simulink model "IOControls"  (R2019b)
settings: configuration reference "ConfigSet_IOControls_Reference" (kept outside this file)
model workspace (MAT data in the model file):
  SampleTime = 0.05
libraries: IOStateMachinesLib x274, SignalGeneratorsLib x1, simulink x1
(part 1 of 10)
settings Model: Creator=lonkaran  LastModifiedBy=bnadpurohit
settings ConfigSetRef: SourceName=ConfigSet_IOControls_Reference  SourceLocation=Base Workspace

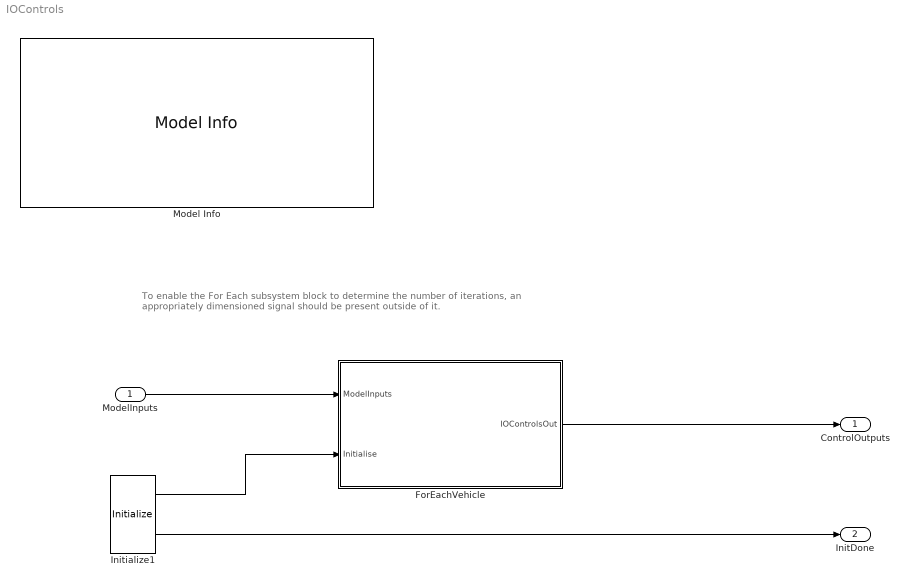
== system IOControls ==
  note: To enable the For Each subsystem block to determine the number of iterations,
      | an appropriately dimensioned signal should be present outside of it.
  ModelInputs : Inport  OutDataTypeStr=Bus: BD_IOControls_In_Vehicle  PortDimensions=MaxVehicles  BusOutputAsStruct=on
  ForEachVehicle : Subsystem  TreatAsAtomicUnit=on
  Initialize1 : SignalGeneratorsLib/Initialize  InitTime=2  SampleTime=0.1
      settings: SourceProductName=Signal Generators
  Model Info : simulink/Model-Wide Utilities/Model Info  Frame=on  DisplayStringWithTags=Model Info\nTemplate Name: IOControlsTemplate\nTemplate Model version number: 1.61\nLast modification date: Thu Jan 23 11:29:17 2020\nModel description:\n\nThis model was created on : %<LastModificationDate> \n automatically by the create_io_controls script using the data available from \nBEML_EMU Model IO.csv  HorizontalTextAlignment=Left  LeftAlignmentValue=0.02
  ControlOutputs : Outport  OutDataTypeStr=Bus: BD_IOControls_Out_Vehicle  VectorParamsAs1DForOutWhenUnconnected=off  BusOutputAsStruct=on
  InitDone : Outport  Port=2  VectorParamsAs1DForOutWhenUnconnected=off
  wires:
  ForEachVehicle/1(IOControlsOut) -> ControlOutputs/1
  ModelInputs/1 -> ForEachVehicle/1(ModelInputs)
  Initialize1/1 -> ForEachVehicle/2(Initialise)
  Initialize1/2 -> InitDone/1

== system IOControls/ForEachVehicle ==
  note: Process inputs from each panel
  ModelInputs : Inport  Partition=on  PartitionDimension=1  PartitionWidth=1  PartitionOffset=0
  Initialise : Inport  Port=2
  For Each : ForEach  DisableCoverage=on
  IOControls : Subsystem
  OutputMapper : Subsystem
  IOControlsOut : Outport  ConcatenationDimension=1  VectorParamsAs1DForOutWhenUnconnected=off
  wires:
  OutputMapper/1(IOControlsOut) -> IOControlsOut/1
  IOControls/1(TierControlsInputs) -> OutputMapper/1(TierControlsInputs)
  ModelInputs/1 -> IOControls/1(ModelInputs)
  Initialise/1 -> IOControls/2(Initialise)
  IOControls/2(TierControlsMCBTrip) -> OutputMapper/2(TierControlsMCBTrip)

== system IOControls/ForEachVehicle/IOControls ==
  ModelInputs : Inport
  Initialise : Inport  Port=2
  BC_Inputs : BusCreator  Inputs=2
  BC_MCBTrip : BusCreator  Inputs=2
  CabControl : Subsystem
  Non-CabControl : Subsystem
  TierControlsInputs : Outport  VectorParamsAs1DForOutWhenUnconnected=off
  TierControlsMCBTrip : Outport  Port=2  VectorParamsAs1DForOutWhenUnconnected=off
  wires:
  BC_Inputs/1 -> TierControlsInputs/1
  BC_MCBTrip/1 -> TierControlsMCBTrip/1
  ModelInputs/1 -> CabControl/1(ModelInputs), Non-CabControl/1(ModelInputs)
  Initialise/1 -> CabControl/2(Initialise), Non-CabControl/2(Initialise)
  CabControl/1(TierControlsInputs) -> BC_Inputs/1
  CabControl/2(TierControlsMCBTrip) -> BC_MCBTrip/1
  Non-CabControl/1(TierControlsInputs) -> BC_Inputs/2
  Non-CabControl/2(TierControlsMCBTrip) -> BC_MCBTrip/2

== system IOControls/ForEachVehicle/OutputMapper ==
  TierControlsInputs : Inport
  TierControlsMCBTrip : Inport  Port=2
  BC_IOControlsOut : BusCreator  Inputs=3  OutDataTypeStr=Bus: BD_IOControls_Out_Vehicle  NonVirtualBus=on
  BS_Inputs : BusSelector  OutputSignals=CabControl.DriverDesk.OperatingPanel1.EmergencyBrakePB,CabControl.DriverDesk.OperatingPanel1.HornPB,CabControl.DriverDesk.OperatingPanel1.CabConsoleLightPB,CabControl.DriverDesk.OperatingPanel1.DoorProvenLoopCutoutPB,CabControl.DriverDesk.OperatingPanel1.LeftDoorClosePBOperatingPanel1,CabControl.DriverDesk.OperatingPanel1.RightDoorClosePBOperatingPanel1,CabControl.DriverDesk.OperatingPanel1.LeftDoorOpenPBOperatingPanel1,CabControl.DriverDesk.OperatingPanel1.RightDoorOpenPBOperatingPanel1,CabControl.DriverDesk.OperatingPanel1.CabMainLightPB,CabControl.DriverDesk.OperatingPanel1.ParkingBrakeOnSwitch,CabControl.DriverDesk.OperatingPanel1.ParkingBrakeOffSwitch,CabControl.DriverDesk.OperatingPanel1.DoorCloseAnnouncementPB,CabControl.DriverDesk.OperatingPanel3.ROSPB,CabControl.DriverDesk.OperatingPanel3.UTOPB,CabControl.DriverDesk.OperatingPanel3.ATOStartPB,CabControl.DriverDesk.OperatingPanel3.EmergencyBrakeResetPB,CabControl.DriverDesk.MasterController.ControlKey,CabControl.DriverDesk.MasterController.ModeSelector,CabControl.DriverDesk.MasterController.MasterControllerHandle,CabControl.DriverDesk.MasterController.DeadmanSafetyDevice,CabControl.DriverDeskLeft.OperatingPanel2.CallOnLightPB,CabControl.DriverDeskLeft.OperatingPanel2.VCBOpenPB,CabControl.DriverDeskLeft.OperatingPanel2.WiperSelectionSwitch,CabControl.DriverDeskLeft.OperatingPanel2.WiperPump,CabControl.DriverDeskLeft.OperatingPanel2.LIMPHomePB,CabControl.DriverDeskLeft.OperatingPanel2.PowerOffPB,CabControl.DriverDeskLeft.OperatingPanel2.PantoDownPB,CabControl.DriverDeskLeft.OperatingPanel2.VCBClosePB,CabControl.DriverDeskLeft.OperatingPanel2.LeftDoorOpenPBOperatingPanel2,CabControl.DriverDeskLeft.OperatingPanel2.LeftDoorOpenPB1OperatingPanel2,CabControl.DriverDeskLeft.OperatingPanel2.LeftDoorClosePBOperatingPanel2,CabControl.DriverDeskLeft.OperatingPanel2.PantoUpPB,CabControl.DriverDeskLeft.OperatingPanel2.SafetyCutoutSS,CabControl.DriverDeskLeft.OperatingPanel2.BrakeLoopCutoutSS,CabControl.DriverDeskLeft.OperatingPanel2.PantoSelector,CabControl.DriverDeskLeft.OperatingPanel2.DeadmanBypassSwitch,CabControl.DriverDeskLeft.OperatingPanel2.HeadLightSwitch,CabControl.DriverDeskRight.OperatingPanel5.UncouplePB,CabControl.DriverDeskRight.OperatingPanel5.FlasherLightPB,CabControl.DriverDeskRight.OperatingPanel5.FloodLightPB,CabControl.DriverDeskRight.OperatingPanel5.BatteryResetPB,CabControl.DriverDeskRight.OperatingPanel5.RightDoorOpenPBOperatingPanel5,CabControl.DriverDeskRight.OperatingPanel5.RightDoorOpenPB1OperatingPanel5,CabControl.DriverDeskRight.OperatingPanel5.RightDoorClosePBOperatingPanel5,CabControl.DriverDeskRight.OperatingPanel5.DoorProvenLoopOutputSwitch,CabControl.DriverDeskRight.OperatingPanel5.LampTestPB,CabControl.DriverDeskRight.OperatingPanel5.WFLTestPB,CabControl.DriverDeskRight.OperatingPanel5.WiperControlSwitch,CabControl.DriverDeskRight.OperatingPanel5.EmergencyStopPB,CabControl.DriverDeskRight.OperatingPanel5.HoldDoorCloseBypassSS,CabControl.DriverDeskRight.OperatingPanel5.CabBoosterFanSS,CabControl.DriverDeskRight.OperatingPanel5.EmergencyBrakePBBypassSS,CabControl.DriversSideCovingPanel.CabEEDLeft,CabControl.Non-driversSideCovingPanel.CabEEDRight,CabControl.EmergencyDoor.SafetyCover,CabControl.EmergencyDoor.DummyCover,CabControl.EmergencyDoor.RampCoverLockingLever,CabControl.EmergencyDoor.RampCover,CabControl.EmergencyDoor.RampHandle,CabControl.EmergencyDoor.RampEndSupport,CabControl.EmergencyDoor.RampMiddleSupport,CabControl.EmergencyDoor.WinderHandlesAccessCover,CabControl.EmergencyDoor.LargeHandle,CabControl.EmergencyDoor.RampWinder,CabControl.EmergencyDoor.SmallHandle,CabControl.EmergencyDoor.EmergencyDoorGasSpring,CabControl.EmergencyDoor.DoorWinder,Non-CabControl.CircuitBreakersofEDB.EBLR2CB,Non-CabControl.CircuitBreakersofEDB.EBMVCB,Non-CabControl.CircuitBreakersofEDB.EDCB,Non-CabControl.CircuitBreakersofEDB.ELCB1,Non-CabControl.CircuitBreakersofEDB.ELCB2,Non-CabControl.CircuitBreakersofEDB.ERCB,Non-CabControl.CircuitBreakersofEDB.HCB,Non-CabControl.CircuitBreakersofEDB.HLLCB,Non-CabControl.CircuitBreakersofEDB.HLRCB,Non-CabControl.CircuitBreakersofEDB.ILCB1,Non-CabControl.CircuitBreakersofEDB.ILCB2,Non-CabControl.CircuitBreakersofEDB.LDICB,Non-CabControl.CircuitBreakersofEDB.LDLCB,Non-CabControl.CircuitBreakersofEDB.LDRCB,Non-CabControl.CircuitBreakersofEDB.MLCB,Non-CabControl.CircuitBreakersofEDB.MMCB,Non-CabControl.CircuitBreakersofEDB.NBCB,Non-CabControl.CircuitBreakersofEDB.NVICB,Non-CabControl.CircuitBreakersofEDB.OCCB1,Non-CabControl.CircuitBreakersofEDB.OCCB2,Non-CabControl.CircuitBreakersofEDB.ODDCB,Non-CabControl.CircuitBreakersofEDB.PBCB,Non-CabControl.CircuitBreakersofEDB.PISCB1,Non-CabControl.CircuitBreakersofEDB.PISCB2,Non-CabControl.CircuitBreakersofEDB.POCB,Non-CabControl.CircuitBreakersofEDB.PPU1CB,Non-CabControl.CircuitBreakersofEDB.PPU2CB,Non-CabControl.CircuitBreakersofEDB.PPU3CB,Non-CabControl.CircuitBreakersofEDB.RIO1CB,Non-CabControl.CircuitBreakersofEDB.RIO2CB,Non-CabControl.CircuitBreakersofEDB.SIOCB1,Non-CabControl.CircuitBreakersofEDB.SIOCB2,Non-CabControl.CircuitBreakersofEDB.SSICB,Non-CabControl.CircuitBreakersofEDB.TBCCB1,Non-CabControl.CircuitBreakersofEDB.TBCCB2,Non-CabControl.CircuitBreakersofEDB.TBNCB,Non-CabControl.CircuitBreakersofEDB.TDICB,Non-CabControl.CircuitBreakersofEDB.TLLCB,Non-CabControl.CircuitBreakersofEDB.TLRCB,Non-CabControl.CircuitBreakersofEDB.TRIVCB,Non-CabControl.CircuitBreakersofEDB.TVDUCB,Non-CabControl.CircuitBreakersofEDB.TWVCB,Non-CabControl.CircuitBreakersofEDB.VCCBOrUCCB,Non-CabControl.CircuitBreakersofEDB.VCBCCB,Non-CabControl.CircuitBreakersofEDB.VIO1CB,Non-CabControl.CircuitBreakersofEDB.VIO2CB,Non-CabControl.CircuitBreakersofEDB.WFLCB,Non-CabControl.CircuitBreakersofEDB.WIFICB,Non-CabControl.CircuitBreakersofEDB.WWCB,Non-CabControl.CircuitBreakersofEDB.BECUCB1,Non-CabControl.CircuitBreakersofEDB.BECUCB2,Non-CabControl.CircuitBreakersofEDB.BECUCB3,Non-CabControl.CircuitBreakersofEDB.RSACB,Non-CabControl.CircuitBreakersofEDB.CMCCB,Non-CabControl.CircuitBreakersofEDB.CILCB,Non-CabControl.CircuitBreakersofEDB.CICB,Non-CabControl.CircuitBreakersofEDB.CELCB,Non-CabControl.CircuitBreakersofEDB.CECB,Non-CabControl.CircuitBreakersofEDB.CDUCB,Non-CabControl.CircuitBreakersofEDB.CCNVIO1CB,Non-CabControl.CircuitBreakersofEDB.CBTCCB1,Non-CabControl.CircuitBreakersofEDB.CBFCCB,Non-CabControl.CircuitBreakersofEDB.CBFCB,Non-CabControl.CircuitBreakersofEDB.C1CB,Non-CabControl.CircuitBreakersofEDB.BLCB,Non-CabControl.CircuitBreakersofEDB.ZVBACB,Non-CabControl.CircuitBreakersofEDB.EBLR1CB,Non-CabControl.CircuitBreakersofEDB.DRCB,Non-CabControl.CircuitBreakersofEDB.DPLCB,Non-CabControl.CircuitBreakersofEDB.DMICB,Non-CabControl.CircuitBreakersofEDB.DLCB,Non-CabControl.CircuitBreakersofEDB.DIOCB2,Non-CabControl.CircuitBreakersofEDB.DIOCB1,Non-CabControl.CircuitBreakersofEDB.CSCCB,Non-CabControl.CircuitBreakersofEDB.CSBCB,Non-CabControl.CircuitBreakersofEDB.CSACB,Non-CabControl.CircuitBreakersofEDB.CRSBCB,Non-CabControl.CircuitBreakersofEDB.SOCB2,Non-CabControl.CircuitBreakersofEDB.SOCB1,Non-CabControl.CircuitBreakersofEDB.MSOCB5,Non-CabControl.CircuitBreakersofEDB.MSOCB4,Non-CabControl.CircuitBreakersofEDB.MSOCB3,Non-CabControl.CircuitBreakersofEDB.MSOCB2,Non-CabControl.CircuitBreakersofEDB.MSOCB1,Non-CabControl.CircuitBreakersofEDB.HVAC1,Non-CabControl.CircuitBreakersofEDB.SAC2CCB,Non-CabControl.CircuitBreakersofEDB.HVAC2,Non-CabControl.CircuitBreakersofEDB.SAC1CCB,Non-CabControl.CircuitBreakersofEDB.CMCB,Non-CabControl.CircuitBreakersofEDB.AC2CB,Non-CabControl.CircuitBreakersofEDB.AC1CB,Non-CabControl.CircuitBreakersofEDB.FDSCB,Non-CabControl.CircuitBreakersofEDB.BCBCB,Non-CabControl.CircuitBreakersofEDB.ERVRCB1,Non-CabControl.CircuitBreakersofEDB.ERVRCB2,Non-CabControl.CircuitBreakersofEDB.ESKCB,Non-CabControl.CircuitBreakersofEDB.HMCB,Non-CabControl.CircuitBreakersofEDB.SP1CB,Non-CabControl.CircuitBreakersofEDB.SP2CB,Non-CabControl.CircuitBreakersofEDB.SP3CB,Non-CabControl.CircuitBreakersofEDB.SP4CB,Non-CabControl.CircuitBreakersofEDB.SP5CB,Non-CabControl.CircuitBreakersofEDB.SPCB6,Non-CabControl.CircuitBreakersofEDB.SPCB7,Non-CabControl.CircuitBreakersofEDB.SPCB8,Non-CabControl.CircuitBreakersofEDB.RPTCB,Non-CabControl.CircuitBreakersofEDB.TERCB1,Non-CabControl.CircuitBreakersofEDB.TERCB2,Non-CabControl.CircuitBreakersofEDB.SPSW,Non-CabControl.CircuitBreakersofEDB.SPPB,Non-CabControl.CircuitBreakersofEDB.APSCB,Non-CabControl.CircuitBreakersofEDB.APSICB,Non-CabControl.CircuitBreakersofEDB.BCGCB,Non-CabControl.CircuitBreakersofEDB.DSCB,Non-CabControl.CircuitBreakersofEDB.MTBMCCB,Non-CabControl.CircuitBreakersofEDB.PADCB,Non-CabControl.CircuitBreakersofEDB.PANCB,Non-CabControl.CircuitBreakersofEDB.SSCB,Non-CabControl.CircuitBreakersofEDB.PTCB,Non-CabControl.CircuitBreakersofEDB.VCBCB,Non-CabControl.CircuitBreakersofEDB.SP12CB,Non-CabControl.CircuitBreakersofEDB.MTBM1CB,Non-CabControl.CircuitBreakersofEDB.MTBM2CB,Non-CabControl.CircuitBreakersofEDB.SP11CB,Non-CabControl.CircuitBreakersofEDB.SP6CB,Non-CabControl.CircuitBreakersofEDB.MTOPCB,Non-CabControl.CircuitBreakersofEDB.ORDCOS,Non-CabControl.CircuitBreakersofEDB.ADDCOS,Non-CabControl.InteriorDoorControls.LeftDoor1DCUCB,Non-CabControl.InteriorDoorControls.LeftDoor2DCUCB,Non-CabControl.InteriorDoorControls.LeftDoor3DCUCB,Non-CabControl.InteriorDoorControls.LeftDoor4DCUCB,Non-CabControl.InteriorDoorControls.RightDoor1DCUCB,Non-CabControl.InteriorDoorControls.RightDoor2DCUCB,Non-CabControl.InteriorDoorControls.RightDoor3DCUCB,Non-CabControl.InteriorDoorControls.RightDoor4DCUCB,Non-CabControl.InteriorDoorControls.LeftDoor1Coving,Non-CabControl.InteriorDoorControls.LeftDoor2Coving,Non-CabControl.InteriorDoorControls.LeftDoor3Coving,Non-CabControl.InteriorDoorControls.LeftDoor4Coving,Non-CabControl.InteriorDoorControls.RightDoor1Coving,Non-CabControl.InteriorDoorControls.RightDoor2Coving,Non-CabControl.InteriorDoorControls.RightDoor3Coving,Non-CabControl.InteriorDoorControls.RightDoor4Coving,Non-CabControl.InteriorDoorControls.LeftDoor1EED,Non-CabControl.InteriorDoorControls.LeftDoor2EED,Non-CabControl.InteriorDoorControls.LeftDoor3EED,Non-CabControl.InteriorDoorControls.LeftDoor4EED,Non-CabControl.InteriorDoorControls.RightDoor1EED,Non-CabControl.InteriorDoorControls.RightDoor2EED,Non-CabControl.InteriorDoorControls.RightDoor3EED,Non-CabControl.InteriorDoorControls.RightDoor4EED,Non-CabControl.InteriorDoorControls.LeftDoor1ManualClose,Non-CabControl.InteriorDoorControls.LeftDoor2ManualClose,Non-CabControl.InteriorDoorControls.LeftDoor3ManualClose,Non-CabControl.InteriorDoorControls.LeftDoor4ManualClose,Non-CabControl.InteriorDoorControls.RightDoor1ManualClose,Non-CabControl.InteriorDoorControls.RightDoor2ManualClose,Non-CabControl.InteriorDoorControls.RightDoor3ManualClose,Non-CabControl.InteriorDoorControls.RightDoor4ManualClose,Non-CabControl.InteriorDoorControls.LeftDoor1ManualOpen,Non-CabControl.InteriorDoorControls.LeftDoor2ManualOpen,Non-CabControl.InteriorDoorControls.LeftDoor3ManualOpen,Non-CabControl.InteriorDoorControls.LeftDoor4ManualOpen,Non-CabControl.InteriorDoorControls.RightDoor1ManualOpen,Non-CabControl.InteriorDoorControls.RightDoor2ManualOpen,Non-CabControl.InteriorDoorControls.RightDoor3ManualOpen,Non-CabControl.InteriorDoorControls.RightDoor4ManualOpen,Non-CabControl.InteriorDoorControls.LeftDoor1Lockout,Non-CabControl.InteriorDoorControls.LeftDoor2Lockout,Non-CabControl.InteriorDoorControls.LeftDoor3Lockout,Non-CabControl.InteriorDoorControls.LeftDoor4Lockout,Non-CabControl.InteriorDoorControls.RightDoor1Lockout,Non-CabControl.InteriorDoorControls.RightDoor2Lockout,Non-CabControl.InteriorDoorControls.RightDoor3Lockout,Non-CabControl.InteriorDoorControls.RightDoor4Lockout,Non-CabControl.ExteriorDoorControls.LeftDoorEADCover,Non-CabControl.ExteriorDoorControls.RightDoorEADCover,Non-CabControl.ExteriorDoorControls.LeftDoorEAD,Non-CabControl.ExteriorDoorControls.RightDoorEAD,Non-CabControl.PneumaticControls.ParkBrakeIsolationCockBogie1,Non-CabControl.PneumaticControls.ParkBrakeIsolationCockBogie2,Non-CabControl.PneumaticControls.MRIsolationCock,Non-CabControl.PneumaticControls.UncouplingCock,Non-CabControl.PneumaticControls.Horn1IsolationCock,Non-CabControl.PneumaticControls.Horn2IsolationCock,Non-CabControl.PneumaticControls.MREPIsolationCockEnd1,Non-CabControl.PneumaticControls.BIC1Inside,Non-CabControl.PneumaticControls.BIC1Outside,Non-CabControl.PneumaticControls.BIC2Inside,Non-CabControl.PneumaticControls.BIC2Outside,Non-CabControl.PneumaticControls.MREPIsolationCockEnd2,Non-CabControl.PneumaticControls.EPIC,Non-CabControl.PneumaticControls.ASCOEnd1,Non-CabControl.PneumaticControls.ASCOEnd2,Non-CabControl.PneumaticControls.ASIsolationCock,Non-CabControl.PneumaticControls.SR,Non-CabControl.PneumaticControls.ParkingBrakeManualReleaseBogie1Handle1,Non-CabControl.PneumaticControls.ParkingBrakeManualReleaseBogie1Handle2,Non-CabControl.PneumaticControls.ParkingBrakeManualReleaseBogie2Handle1,Non-CabControl.PneumaticControls.ParkingBrakeManualReleaseBogie2Handle2,Non-CabControl.PassengerEmergencyControlUnit.PECUPushButton,Non-CabControl.PassengerEmergencyControlUnit.Microphone,Non-CabControl.PassengerEmergencyControlUnit.DriversBackDoor,Non-CabControl.EDBPanel.PantographIsolationCock,Non-CabControl.EDBPanel.VCBIsolationCock,Non-CabControl.EDBPanel.ORDPlunger  OutputAsBus=on
  BS_MCBTrip : BusSelector  OutputSignals=Non-CabControl.CircuitBreakersofEDB.EBLR2CB,Non-CabControl.CircuitBreakersofEDB.EBMVCB,Non-CabControl.CircuitBreakersofEDB.EDCB,Non-CabControl.CircuitBreakersofEDB.ELCB1,Non-CabControl.CircuitBreakersofEDB.ELCB2,Non-CabControl.CircuitBreakersofEDB.ERCB,Non-CabControl.CircuitBreakersofEDB.HCB,Non-CabControl.CircuitBreakersofEDB.HLLCB,Non-CabControl.CircuitBreakersofEDB.HLRCB,Non-CabControl.CircuitBreakersofEDB.ILCB1,Non-CabControl.CircuitBreakersofEDB.ILCB2,Non-CabControl.CircuitBreakersofEDB.LDICB,Non-CabControl.CircuitBreakersofEDB.LDLCB,Non-CabControl.CircuitBreakersofEDB.LDRCB,Non-CabControl.CircuitBreakersofEDB.MLCB,Non-CabControl.CircuitBreakersofEDB.MMCB,Non-CabControl.CircuitBreakersofEDB.NBCB,Non-CabControl.CircuitBreakersofEDB.NVICB,Non-CabControl.CircuitBreakersofEDB.OCCB1,Non-CabControl.CircuitBreakersofEDB.OCCB2,Non-CabControl.CircuitBreakersofEDB.ODDCB,Non-CabControl.CircuitBreakersofEDB.PBCB,Non-CabControl.CircuitBreakersofEDB.PISCB1,Non-CabControl.CircuitBreakersofEDB.PISCB2,Non-CabControl.CircuitBreakersofEDB.POCB,Non-CabControl.CircuitBreakersofEDB.PPU1CB,Non-CabControl.CircuitBreakersofEDB.PPU2CB,Non-CabControl.CircuitBreakersofEDB.PPU3CB,Non-CabControl.CircuitBreakersofEDB.RIO1CB,Non-CabControl.CircuitBreakersofEDB.RIO2CB,Non-CabControl.CircuitBreakersofEDB.SIOCB1,Non-CabControl.CircuitBreakersofEDB.SIOCB2,Non-CabControl.CircuitBreakersofEDB.SSICB,Non-CabControl.CircuitBreakersofEDB.TBCCB1,Non-CabControl.CircuitBreakersofEDB.TBCCB2,Non-CabControl.CircuitBreakersofEDB.TBNCB,Non-CabControl.CircuitBreakersofEDB.TDICB,Non-CabControl.CircuitBreakersofEDB.TLLCB,Non-CabControl.CircuitBreakersofEDB.TLRCB,Non-CabControl.CircuitBreakersofEDB.TRIVCB,Non-CabControl.CircuitBreakersofEDB.TVDUCB,Non-CabControl.CircuitBreakersofEDB.TWVCB,Non-CabControl.CircuitBreakersofEDB.VCCBOrUCCB,Non-CabControl.CircuitBreakersofEDB.VCBCCB,Non-CabControl.CircuitBreakersofEDB.VIO1CB,Non-CabControl.CircuitBreakersofEDB.VIO2CB,Non-CabControl.CircuitBreakersofEDB.WFLCB,Non-CabControl.CircuitBreakersofEDB.WIFICB,Non-CabControl.CircuitBreakersofEDB.WWCB,Non-CabControl.CircuitBreakersofEDB.BECUCB1,Non-CabControl.CircuitBreakersofEDB.BECUCB2,Non-CabControl.CircuitBreakersofEDB.BECUCB3,Non-CabControl.CircuitBreakersofEDB.RSACB,Non-CabControl.CircuitBreakersofEDB.CMCCB,Non-CabControl.CircuitBreakersofEDB.CILCB,Non-CabControl.CircuitBreakersofEDB.CICB,Non-CabControl.CircuitBreakersofEDB.CELCB,Non-CabControl.CircuitBreakersofEDB.CECB,Non-CabControl.CircuitBreakersofEDB.CDUCB,Non-CabControl.CircuitBreakersofEDB.CCNVIO1CB,Non-CabControl.CircuitBreakersofEDB.CBTCCB1,Non-CabControl.CircuitBreakersofEDB.CBFCCB,Non-CabControl.CircuitBreakersofEDB.CBFCB,Non-CabControl.CircuitBreakersofEDB.C1CB,Non-CabControl.CircuitBreakersofEDB.BLCB,Non-CabControl.CircuitBreakersofEDB.ZVBACB,Non-CabControl.CircuitBreakersofEDB.EBLR1CB,Non-CabControl.CircuitBreakersofEDB.DRCB,Non-CabControl.CircuitBreakersofEDB.DPLCB,Non-CabControl.CircuitBreakersofEDB.DMICB,Non-CabControl.CircuitBreakersofEDB.DLCB,Non-CabControl.CircuitBreakersofEDB.DIOCB2,Non-CabControl.CircuitBreakersofEDB.DIOCB1,Non-CabControl.CircuitBreakersofEDB.CSCCB,Non-CabControl.CircuitBreakersofEDB.CSBCB,Non-CabControl.CircuitBreakersofEDB.CSACB,Non-CabControl.CircuitBreakersofEDB.CRSBCB,Non-CabControl.CircuitBreakersofEDB.SOCB2,Non-CabControl.CircuitBreakersofEDB.SOCB1,Non-CabControl.CircuitBreakersofEDB.MSOCB5,Non-CabControl.CircuitBreakersofEDB.MSOCB4,Non-CabControl.CircuitBreakersofEDB.MSOCB3,Non-CabControl.CircuitBreakersofEDB.MSOCB2,Non-CabControl.CircuitBreakersofEDB.MSOCB1,Non-CabControl.CircuitBreakersofEDB.HVAC1,Non-CabControl.CircuitBreakersofEDB.SAC2CCB,Non-CabControl.CircuitBreakersofEDB.HVAC2,Non-CabControl.CircuitBreakersofEDB.SAC1CCB,Non-CabControl.CircuitBreakersofEDB.CMCB,Non-CabControl.CircuitBreakersofEDB.AC2CB,Non-CabControl.CircuitBreakersofEDB.AC1CB,Non-CabControl.CircuitBreakersofEDB.FDSCB,Non-CabControl.CircuitBreakersofEDB.BCBCB,Non-CabControl.CircuitBreakersofEDB.ERVRCB1,Non-CabControl.CircuitBreakersofEDB.ERVRCB2,Non-CabControl.CircuitBreakersofEDB.ESKCB,Non-CabControl.CircuitBreakersofEDB.HMCB,Non-CabControl.CircuitBreakersofEDB.SP1CB,Non-CabControl.CircuitBreakersofEDB.SP2CB,Non-CabControl.CircuitBreakersofEDB.SP3CB,Non-CabControl.CircuitBreakersofEDB.SP4CB,Non-CabControl.CircuitBreakersofEDB.SP5CB,Non-CabControl.CircuitBreakersofEDB.SPCB6,Non-CabControl.CircuitBreakersofEDB.SPCB7,Non-CabControl.CircuitBreakersofEDB.SPCB8,Non-CabControl.CircuitBreakersofEDB.RPTCB,Non-CabControl.CircuitBreakersofEDB.TERCB1,Non-CabControl.CircuitBreakersofEDB.TERCB2,Non-CabControl.CircuitBreakersofEDB.APSCB,Non-CabControl.CircuitBreakersofEDB.APSICB,Non-CabControl.CircuitBreakersofEDB.BCGCB,Non-CabControl.CircuitBreakersofEDB.DSCB,Non-CabControl.CircuitBreakersofEDB.MTBMCCB,Non-CabControl.CircuitBreakersofEDB.PADCB,Non-CabControl.CircuitBreakersofEDB.PANCB,Non-CabControl.CircuitBreakersofEDB.SSCB,Non-CabControl.CircuitBreakersofEDB.PTCB,Non-CabControl.CircuitBreakersofEDB.VCBCB,Non-CabControl.CircuitBreakersofEDB.SP12CB,Non-CabControl.CircuitBreakersofEDB.MTBM1CB,Non-CabControl.CircuitBreakersofEDB.MTBM2CB,Non-CabControl.CircuitBreakersofEDB.SP11CB,Non-CabControl.CircuitBreakersofEDB.SP6CB,Non-CabControl.CircuitBreakersofEDB.MTOPCB,Non-CabControl.InteriorDoorControls.LeftDoor1DCUCB,Non-CabControl.InteriorDoorControls.LeftDoor2DCUCB,Non-CabControl.InteriorDoorControls.LeftDoor3DCUCB,Non-CabControl.InteriorDoorControls.LeftDoor4DCUCB,Non-CabControl.InteriorDoorControls.RightDoor1DCUCB,Non-CabControl.InteriorDoorControls.RightDoor2DCUCB,Non-CabControl.InteriorDoorControls.RightDoor3DCUCB,Non-CabControl.InteriorDoorControls.RightDoor4DCUCB  OutputAsBus=on
  OutputStates : Constant  Value=0  OutDataTypeStr=Bus: BD_IOControls_Out_Vehicle_OutputStates
  IOControlsOut : Outport  VectorParamsAs1DForOutWhenUnconnected=off
  wires:
  BC_IOControlsOut/1 -> IOControlsOut/1  "IOControls"
  OutputStates/1 -> BC_IOControlsOut/3  "OutputStates"
  TierControlsInputs/1 -> BS_Inputs/1
  BS_Inputs/1 -> BC_IOControlsOut/1  "InputStates"
  TierControlsMCBTrip/1 -> BS_MCBTrip/1
  BS_MCBTrip/1 -> BC_IOControlsOut/2  "MCBTripStates"

== system IOControls/ForEachVehicle/IOControls/CabControl ==
  ModelInputs : Inport
  Initialise : Inport  Port=2
  BC_Inputs : BusCreator  Inputs=6
  BC_MCBTrip : BusCreator  Inputs=6
  DriverDesk : Subsystem
  DriverDeskLeft : Subsystem
  DriverDeskRight : Subsystem
  DriversSideCovingPanel : Subsystem
  EmergencyDoor : Subsystem
  Non-driversSideCovingPanel : Subsystem
  TierControlsInputs : Outport  VectorParamsAs1DForOutWhenUnconnected=off
  TierControlsMCBTrip : Outport  Port=2  VectorParamsAs1DForOutWhenUnconnected=off
  wires:
  BC_MCBTrip/1 -> TierControlsMCBTrip/1  "CabControl"
  BC_Inputs/1 -> TierControlsInputs/1  "CabControl"
  ModelInputs/1 -> DriverDesk/1(ModelInputs), DriverDeskLeft/1(ModelInputs), DriverDeskRight/1(ModelInputs), DriversSideCovingPanel/1(ModelInputs), Non-driversSideCovingPanel/1(ModelInputs), EmergencyDoor/1(ModelInputs)
  Initialise/1 -> DriverDesk/2(Initialise), DriverDeskLeft/2(Initialise), DriverDeskRight/2(Initialise), DriversSideCovingPanel/2(Initialise), Non-driversSideCovingPanel/2(Initialise), EmergencyDoor/2(Initialise)
  DriverDesk/1(TierControlsInputs) -> BC_Inputs/1
  DriverDesk/2(TierControlsMCBTrip) -> BC_MCBTrip/1
  DriverDeskLeft/1(TierControlsInputs) -> BC_Inputs/2
  DriverDeskLeft/2(TierControlsMCBTrip) -> BC_MCBTrip/2
  DriverDeskRight/1(TierControlsInputs) -> BC_Inputs/3
  DriverDeskRight/2(TierControlsMCBTrip) -> BC_MCBTrip/3
  DriversSideCovingPanel/1(TierControlsInputs) -> BC_Inputs/4
  DriversSideCovingPanel/2(TierControlsMCBTrip) -> BC_MCBTrip/4
  Non-driversSideCovingPanel/1(TierControlsInputs) -> BC_Inputs/5
  Non-driversSideCovingPanel/2(TierControlsMCBTrip) -> BC_MCBTrip/5
  EmergencyDoor/1(TierControlsInputs) -> BC_Inputs/6
  EmergencyDoor/2(TierControlsMCBTrip) -> BC_MCBTrip/6

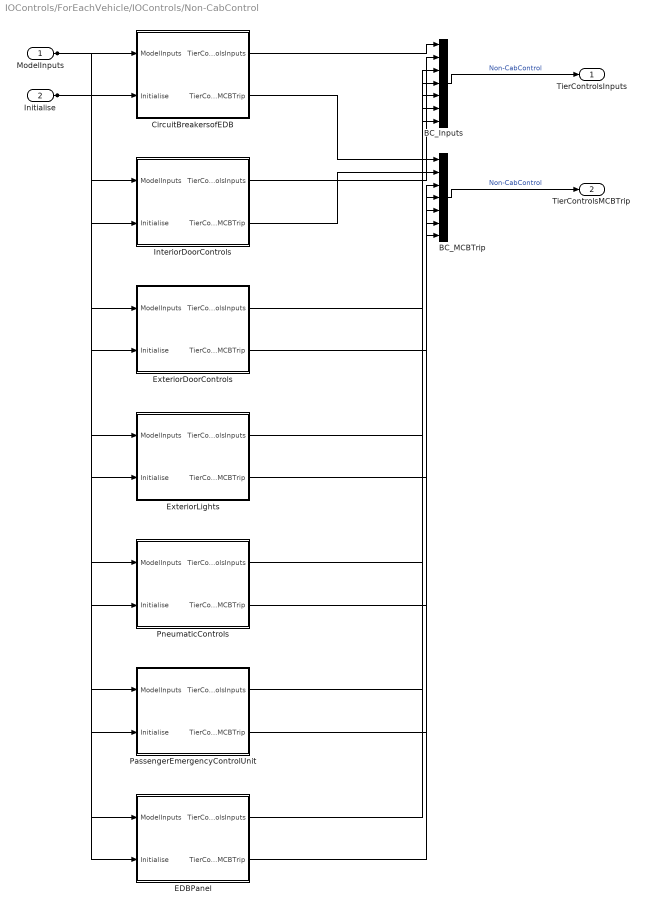
== system IOControls/ForEachVehicle/IOControls/Non-CabControl ==
  ModelInputs : Inport
  Initialise : Inport  Port=2
  BC_Inputs : BusCreator  Inputs=7
  BC_MCBTrip : BusCreator  Inputs=7
  CircuitBreakersofEDB : Subsystem
  EDBPanel : Subsystem
  ExteriorDoorControls : Subsystem
  ExteriorLights : Subsystem
  InteriorDoorControls : Subsystem
  PassengerEmergencyControlUnit : Subsystem
  PneumaticControls : Subsystem
  TierControlsInputs : Outport  VectorParamsAs1DForOutWhenUnconnected=off
  TierControlsMCBTrip : Outport  Port=2  VectorParamsAs1DForOutWhenUnconnected=off
  wires:
  BC_MCBTrip/1 -> TierControlsMCBTrip/1  "Non-CabControl"
  BC_Inputs/1 -> TierControlsInputs/1  "Non-CabControl"
  ModelInputs/1 -> CircuitBreakersofEDB/1(ModelInputs), InteriorDoorControls/1(ModelInputs), ExteriorDoorControls/1(ModelInputs), ExteriorLights/1(ModelInputs), PneumaticControls/1(ModelInputs), PassengerEmergencyControlUnit/1(ModelInputs), EDBPanel/1(ModelInputs)
  Initialise/1 -> CircuitBreakersofEDB/2(Initialise), InteriorDoorControls/2(Initialise), ExteriorDoorControls/2(Initialise), ExteriorLights/2(Initialise), PneumaticControls/2(Initialise), PassengerEmergencyControlUnit/2(Initialise), EDBPanel/2(Initialise)
  CircuitBreakersofEDB/1(TierControlsInputs) -> BC_Inputs/1
  CircuitBreakersofEDB/2(TierControlsMCBTrip) -> BC_MCBTrip/1
  InteriorDoorControls/1(TierControlsInputs) -> BC_Inputs/2
  InteriorDoorControls/2(TierControlsMCBTrip) -> BC_MCBTrip/2
  ExteriorDoorControls/1(TierControlsInputs) -> BC_Inputs/3
  ExteriorDoorControls/2(TierControlsMCBTrip) -> BC_MCBTrip/3
  ExteriorLights/1(TierControlsInputs) -> BC_Inputs/4
  ExteriorLights/2(TierControlsMCBTrip) -> BC_MCBTrip/4
  PneumaticControls/1(TierControlsInputs) -> BC_Inputs/5
  PneumaticControls/2(TierControlsMCBTrip) -> BC_MCBTrip/5
  PassengerEmergencyControlUnit/1(TierControlsInputs) -> BC_Inputs/6
  PassengerEmergencyControlUnit/2(TierControlsMCBTrip) -> BC_MCBTrip/6
  EDBPanel/1(TierControlsInputs) -> BC_Inputs/7
  EDBPanel/2(TierControlsMCBTrip) -> BC_MCBTrip/7

== system IOControls/ForEachVehicle/IOControls/CabControl/DriverDesk ==
  ModelInputs : Inport
  Initialise : Inport  Port=2
  BC_Inputs : BusCreator  Inputs=4
  BC_MCBTrip : BusCreator  Inputs=4
  Gauges : Subsystem
  MasterController : Subsystem
  OperatingPanel1 : Subsystem
  OperatingPanel3 : Subsystem
  TierControlsInputs : Outport  VectorParamsAs1DForOutWhenUnconnected=off
  TierControlsMCBTrip : Outport  Port=2  VectorParamsAs1DForOutWhenUnconnected=off
  wires:
  BC_MCBTrip/1 -> TierControlsMCBTrip/1  "DriverDesk"
  BC_Inputs/1 -> TierControlsInputs/1  "DriverDesk"
  ModelInputs/1 -> OperatingPanel1/1(ModelInputs), OperatingPanel3/1(ModelInputs), Gauges/1(ModelInputs), MasterController/1(ModelInputs)
  Initialise/1 -> OperatingPanel1/2(Initialise), OperatingPanel3/2(Initialise), Gauges/2(Initialise), MasterController/2(Initialise)
  OperatingPanel1/1(TierControlsInputs) -> BC_Inputs/1
  OperatingPanel1/2(TierControlsMCBTrip) -> BC_MCBTrip/1
  OperatingPanel3/1(TierControlsInputs) -> BC_Inputs/2
  OperatingPanel3/2(TierControlsMCBTrip) -> BC_MCBTrip/2
  Gauges/1(TierControlsInputs) -> BC_Inputs/3
  Gauges/2(TierControlsMCBTrip) -> BC_MCBTrip/3
  MasterController/1(TierControlsInputs) -> BC_Inputs/4
  MasterController/2(TierControlsMCBTrip) -> BC_MCBTrip/4

== system IOControls/ForEachVehicle/IOControls/CabControl/DriverDeskLeft ==
  ModelInputs : Inport
  Initialise : Inport  Port=2
  BC_Inputs : BusCreator  Inputs=2
  BC_MCBTrip : BusCreator  Inputs=2
  OperatingPanel2 : Subsystem
  OperatingPanel4 : Subsystem
  TierControlsInputs : Outport  VectorParamsAs1DForOutWhenUnconnected=off
  TierControlsMCBTrip : Outport  Port=2  VectorParamsAs1DForOutWhenUnconnected=off
  wires:
  BC_MCBTrip/1 -> TierControlsMCBTrip/1  "DriverDeskLeft"
  BC_Inputs/1 -> TierControlsInputs/1  "DriverDeskLeft"
  ModelInputs/1 -> OperatingPanel2/1(ModelInputs), OperatingPanel4/1(ModelInputs)
  Initialise/1 -> OperatingPanel2/2(Initialise), OperatingPanel4/2(Initialise)
  OperatingPanel2/1(TierControlsInputs) -> BC_Inputs/1
  OperatingPanel2/2(TierControlsMCBTrip) -> BC_MCBTrip/1
  OperatingPanel4/1(TierControlsInputs) -> BC_Inputs/2
  OperatingPanel4/2(TierControlsMCBTrip) -> BC_MCBTrip/2

== system IOControls/ForEachVehicle/IOControls/CabControl/DriverDeskRight ==
  ModelInputs : Inport
  Initialise : Inport  Port=2
  BC_Inputs : BusCreator  Inputs=1
  BC_MCBTrip : BusCreator  Inputs=1
  OperatingPanel5 : Subsystem
  TierControlsInputs : Outport  VectorParamsAs1DForOutWhenUnconnected=off
  TierControlsMCBTrip : Outport  Port=2  VectorParamsAs1DForOutWhenUnconnected=off
  wires:
  BC_MCBTrip/1 -> TierControlsMCBTrip/1  "DriverDeskRight"
  BC_Inputs/1 -> TierControlsInputs/1  "DriverDeskRight"
  ModelInputs/1 -> OperatingPanel5/1(ModelInputs)
  Initialise/1 -> OperatingPanel5/2(Initialise)
  OperatingPanel5/1(TierControlsInputs) -> BC_Inputs/1
  OperatingPanel5/2(TierControlsMCBTrip) -> BC_MCBTrip/1

== system IOControls/ForEachVehicle/IOControls/CabControl/DriversSideCovingPanel ==
  ModelInputs : Inport
  Initialise : Inport  Port=2
  BC_Inputs : BusCreator  Inputs=1
  BC_MCBTrip : BusCreator  Inputs=1
  BS_Control1 : BusSelector  OutputSignals=CabEEDLeft
  CabEEDLeft : Subsystem  mask{InitState=0, ControlStates=[0,1], OnStateValue=1, OffStateValue=0}
      mask prompts: InitState "Initial State"; ControlStates "Software State Values"; OnStateValue "On State Value"; OffStateValue "Off State Value"
  MCBTripGround : Ground
  TierControlsInputs : Outport  VectorParamsAs1DForOutWhenUnconnected=off
  TierControlsMCBTrip : Outport  Port=2  VectorParamsAs1DForOutWhenUnconnected=off
  wires:
  MCBTripGround/1 -> BC_MCBTrip/1
  BC_MCBTrip/1 -> TierControlsMCBTrip/1  "DriversSideCovingPanel"
  BC_Inputs/1 -> TierControlsInputs/1  "DriversSideCovingPanel"
  ModelInputs/1 -> BS_Control1/1
  BS_Control1/1 -> CabEEDLeft/1(InputControl)  "<CabEEDLeft>"
  Initialise/1 -> CabEEDLeft/2(Initialise)
  CabEEDLeft/1(InputState) -> BC_Inputs/1  "CabEEDLeft"

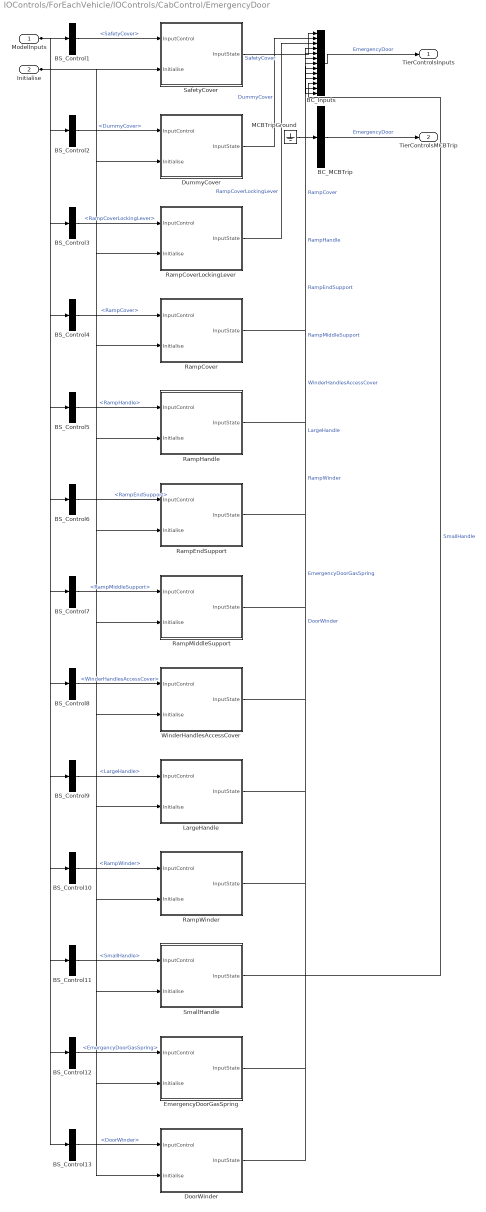
== system IOControls/ForEachVehicle/IOControls/CabControl/EmergencyDoor ==
  ModelInputs : Inport
  Initialise : Inport  Port=2
  BC_Inputs : BusCreator  Inputs=13
  BC_MCBTrip : BusCreator  Inputs=1
  BS_Control1 : BusSelector  OutputSignals=SafetyCover
  BS_Control10 : BusSelector  OutputSignals=RampWinder
  BS_Control11 : BusSelector  OutputSignals=SmallHandle
  BS_Control12 : BusSelector  OutputSignals=EmergencyDoorGasSpring
  BS_Control13 : BusSelector  OutputSignals=DoorWinder
  BS_Control2 : BusSelector  OutputSignals=DummyCover
  BS_Control3 : BusSelector  OutputSignals=RampCoverLockingLever
  BS_Control4 : BusSelector  OutputSignals=RampCover
  BS_Control5 : BusSelector  OutputSignals=RampHandle
  BS_Control6 : BusSelector  OutputSignals=RampEndSupport
  BS_Control7 : BusSelector  OutputSignals=RampMiddleSupport
  BS_Control8 : BusSelector  OutputSignals=WinderHandlesAccessCover
  BS_Control9 : BusSelector  OutputSignals=LargeHandle
  DoorWinder : Subsystem  mask{InitState=0, ControlStates=[0,1,2,3,4,5,6,7,8,9,10,11,12], OnStateValue=12, OffStateValue=0}
      mask prompts: InitState "Initial State"; ControlStates "Software State Values"; OnStateValue "On State Value"; OffStateValue "Off State Value"
  DummyCover : Subsystem  mask{InitState=0, ControlStates=[0,1], OnStateValue=1, OffStateValue=0}
      mask prompts: InitState "Initial State"; ControlStates "Software State Values"; OnStateValue "On State Value"; OffStateValue "Off State Value"
  EmergencyDoorGasSpring : Subsystem  mask{InitState=0, ControlStates=[0,1], OnStateValue=1, OffStateValue=0}
      mask prompts: InitState "Initial State"; ControlStates "Software State Values"; OnStateValue "On State Value"; OffStateValue "Off State Value"
  LargeHandle : Subsystem  mask{InitState=0, ControlStates=[0,1], OnStateValue=1, OffStateValue=0}
      mask prompts: InitState "Initial State"; ControlStates "Software State Values"; OnStateValue "On State Value"; OffStateValue "Off State Value"
  MCBTripGround : Ground
  RampCover : Subsystem  mask{InitState=0, ControlStates=[0,1], OnStateValue=1, OffStateValue=0}
      mask prompts: InitState "Initial State"; ControlStates "Software State Values"; OnStateValue "On State Value"; OffStateValue "Off State Value"
  RampCoverLockingLever : Subsystem  mask{InitState=0, ControlStates=[0,1], OnStateValue=1, OffStateValue=0}
      mask prompts: InitState "Initial State"; ControlStates "Software State Values"; OnStateValue "On State Value"; OffStateValue "Off State Value"
  RampEndSupport : Subsystem  mask{InitState=0, ControlStates=[0,1], OnStateValue=1, OffStateValue=0}
      mask prompts: InitState "Initial State"; ControlStates "Software State Values"; OnStateValue "On State Value"; OffStateValue "Off State Value"
  RampHandle : Subsystem  mask{InitState=0, ControlStates=[0,1], OnStateValue=1, OffStateValue=0}
      mask prompts: InitState "Initial State"; ControlStates "Software State Values"; OnStateValue "On State Value"; OffStateValue "Off State Value"
  RampMiddleSupport : Subsystem  mask{InitState=0, ControlStates=[0,1], OnStateValue=1, OffStateValue=0}
      mask prompts: InitState "Initial State"; ControlStates "Software State Values"; OnStateValue "On State Value"; OffStateValue "Off State Value"
  RampWinder : Subsystem  mask{InitState=0, ControlStates=[0,1,2,3,4,5,6,7,8,9,10,11,12], OnStateValue=12, OffStateValue=0}
      mask prompts: InitState "Initial State"; ControlStates "Software State Values"; OnStateValue "On State Value"; OffStateValue "Off State Value"
  SafetyCover : Subsystem  mask{InitState=0, ControlStates=[0,1], OnStateValue=1, OffStateValue=0}
      mask prompts: InitState "Initial State"; ControlStates "Software State Values"; OnStateValue "On State Value"; OffStateValue "Off State Value"
  SmallHandle : Subsystem  mask{InitState=0, ControlStates=[0,1], OnStateValue=1, OffStateValue=0}
      mask prompts: InitState "Initial State"; ControlStates "Software State Values"; OnStateValue "On State Value"; OffStateValue "Off State Value"
  WinderHandlesAccessCover : Subsystem  mask{InitState=0, ControlStates=[0,1], OnStateValue=1, OffStateValue=0}
      mask prompts: InitState "Initial State"; ControlStates "Software State Values"; OnStateValue "On State Value"; OffStateValue "Off State Value"
  TierControlsInputs : Outport  VectorParamsAs1DForOutWhenUnconnected=off
  TierControlsMCBTrip : Outport  Port=2  VectorParamsAs1DForOutWhenUnconnected=off
  wires:
  MCBTripGround/1 -> BC_MCBTrip/1
  BC_MCBTrip/1 -> TierControlsMCBTrip/1  "EmergencyDoor"
  BC_Inputs/1 -> TierControlsInputs/1  "EmergencyDoor"
  ModelInputs/1 -> BS_Control1/1, BS_Control2/1, BS_Control3/1, BS_Control4/1, BS_Control5/1, BS_Control6/1, BS_Control7/1, BS_Control8/1, BS_Control9/1, BS_Control10/1, BS_Control11/1, BS_Control12/1, BS_Control13/1
  BS_Control1/1 -> SafetyCover/1(InputControl)  "<SafetyCover>"
  Initialise/1 -> SafetyCover/2(Initialise), DummyCover/2(Initialise), RampCoverLockingLever/2(Initialise), RampCover/2(Initialise), RampHandle/2(Initialise), RampEndSupport/2(Initialise), RampMiddleSupport/2(Initialise), WinderHandlesAccessCover/2(Initialise), LargeHandle/2(Initialise), RampWinder/2(Initialise), SmallHandle/2(Initialise), EmergencyDoorGasSpring/2(Initialise), DoorWinder/2(Initialise)
  SafetyCover/1(InputState) -> BC_Inputs/1  "SafetyCover"
  BS_Control2/1 -> DummyCover/1(InputControl)  "<DummyCover>"
  DummyCover/1(InputState) -> BC_Inputs/2  "DummyCover"
  BS_Control3/1 -> RampCoverLockingLever/1(InputControl)  "<RampCoverLockingLever>"
  RampCoverLockingLever/1(InputState) -> BC_Inputs/3  "RampCoverLockingLever"
  BS_Control4/1 -> RampCover/1(InputControl)  "<RampCover>"
  RampCover/1(InputState) -> BC_Inputs/4  "RampCover"
  BS_Control5/1 -> RampHandle/1(InputControl)  "<RampHandle>"
  RampHandle/1(InputState) -> BC_Inputs/5  "RampHandle"
  BS_Control6/1 -> RampEndSupport/1(InputControl)  "<RampEndSupport>"
  RampEndSupport/1(InputState) -> BC_Inputs/6  "RampEndSupport"
  BS_Control7/1 -> RampMiddleSupport/1(InputControl)  "<RampMiddleSupport>"
  RampMiddleSupport/1(InputState) -> BC_Inputs/7  "RampMiddleSupport"
  BS_Control8/1 -> WinderHandlesAccessCover/1(InputControl)  "<WinderHandlesAccessCover>"
  WinderHandlesAccessCover/1(InputState) -> BC_Inputs/8  "WinderHandlesAccessCover"
  BS_Control9/1 -> LargeHandle/1(InputControl)  "<LargeHandle>"
  LargeHandle/1(InputState) -> BC_Inputs/9  "LargeHandle"
  BS_Control10/1 -> RampWinder/1(InputControl)  "<RampWinder>"
  RampWinder/1(InputState) -> BC_Inputs/10  "RampWinder"
  BS_Control11/1 -> SmallHandle/1(InputControl)  "<SmallHandle>"
  SmallHandle/1(InputState) -> BC_Inputs/11  "SmallHandle"
  BS_Control12/1 -> EmergencyDoorGasSpring/1(InputControl)  "<EmergencyDoorGasSpring>"
  EmergencyDoorGasSpring/1(InputState) -> BC_Inputs/12  "EmergencyDoorGasSpring"
  BS_Control13/1 -> DoorWinder/1(InputControl)  "<DoorWinder>"
  DoorWinder/1(InputState) -> BC_Inputs/13  "DoorWinder"

== system IOControls/ForEachVehicle/IOControls/CabControl/Non-driversSideCovingPanel ==
  ModelInputs : Inport
  Initialise : Inport  Port=2
  BC_Inputs : BusCreator  Inputs=1
  BC_MCBTrip : BusCreator  Inputs=1
  BS_Control1 : BusSelector  OutputSignals=CabEEDRight
  CabEEDRight : Subsystem  mask{InitState=0, ControlStates=[0,1], OnStateValue=1, OffStateValue=0}
      mask prompts: InitState "Initial State"; ControlStates "Software State Values"; OnStateValue "On State Value"; OffStateValue "Off State Value"
  MCBTripGround : Ground
  TierControlsInputs : Outport  VectorParamsAs1DForOutWhenUnconnected=off
  TierControlsMCBTrip : Outport  Port=2  VectorParamsAs1DForOutWhenUnconnected=off
  wires:
  MCBTripGround/1 -> BC_MCBTrip/1
  BC_MCBTrip/1 -> TierControlsMCBTrip/1  "Non-driversSideCovingPanel"
  BC_Inputs/1 -> TierControlsInputs/1  "Non-driversSideCovingPanel"
  ModelInputs/1 -> BS_Control1/1
  BS_Control1/1 -> CabEEDRight/1(InputControl)  "<CabEEDRight>"
  Initialise/1 -> CabEEDRight/2(Initialise)
  CabEEDRight/1(InputState) -> BC_Inputs/1  "CabEEDRight"
